simulink model "test"  (R2021a)
settings: Solver=VariableStepAuto  StartTime=0.0  StopTime=10.0  RelTol=1e-3
libraries: c2xlib x9
settings Model: EnablePacing=on  Creator=User  LastModifiedBy=User

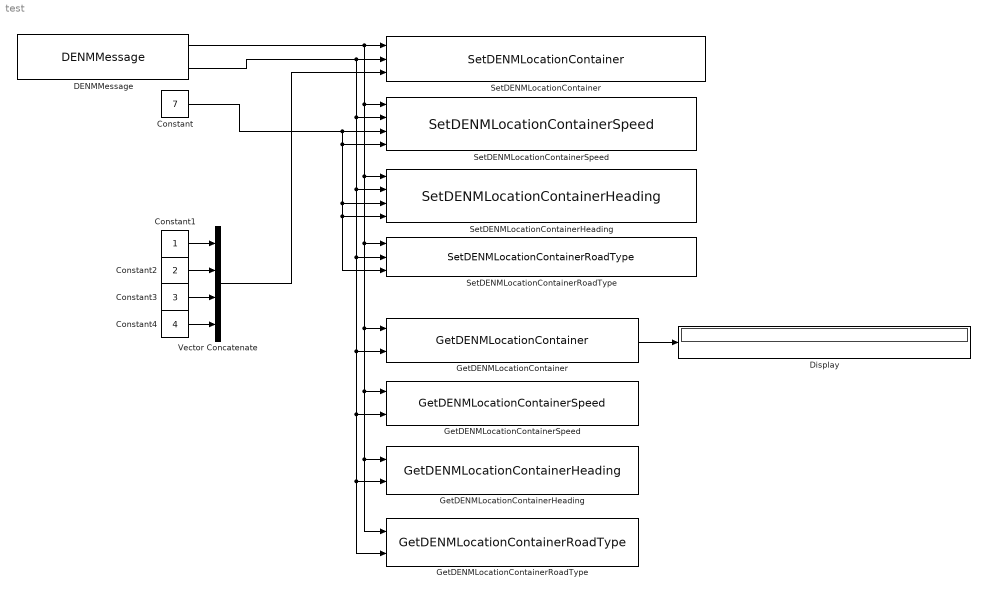
== system test ==
  Constant : Constant  Value=7
  Constant1 : Constant
  Constant2 : Constant  Value=2
  Constant3 : Constant  Value=3
  Constant4 : Constant  Value=4
  DENMMessage : c2xlib/DENMMessage  StationID=1  SequenceNumber=1  SimulateUsing=Code generation
      settings: SourceProductName=C2XLib
  Display : Display
  GetDENMLocationContainer : c2xlib/GetDENMLocationContainer  NumberTraces=1  TraceLength=1  SimulateUsing=Code generation
      settings: SourceProductName=C2XLib
  GetDENMLocationContainerHeading : c2xlib/GetDENMLocationContainerHeading  SimulateUsing=Code generation
      settings: SourceProductName=C2XLib
  GetDENMLocationContainerRoadType : c2xlib/GetDENMLocationContainerRoadType  SimulateUsing=Code generation
      settings: SourceProductName=C2XLib
  GetDENMLocationContainerSpeed : c2xlib/GetDENMLocationContainerSpeed  SimulateUsing=Code generation
      settings: SourceProductName=C2XLib
  SetDENMLocationContainer : c2xlib/SetDENMLocationContainer  NumberTraces=1  SimulateUsing=Code generation
      settings: SourceProductName=C2XLib
  SetDENMLocationContainerHeading : c2xlib/SetDENMLocationContainerHeading  SimulateUsing=Code generation
      settings: SourceProductName=C2XLib
  SetDENMLocationContainerRoadType : c2xlib/SetDENMLocationContainerRoadType  SimulateUsing=Code generation
      settings: SourceProductName=C2XLib
  SetDENMLocationContainerSpeed : c2xlib/SetDENMLocationContainerSpeed  SimulateUsing=Code generation
      settings: SourceProductName=C2XLib
  Vector Concatenate : Concatenate  NumInputs=4
  wires:
  Constant4/1 -> Vector Concatenate/4
  Constant3/1 -> Vector Concatenate/3
  Constant2/1 -> Vector Concatenate/2
  Constant1/1 -> Vector Concatenate/1
  DENMMessage/2 -> SetDENMLocationContainer/2, GetDENMLocationContainer/2, GetDENMLocationContainerSpeed/2, GetDENMLocationContainerRoadType/2, GetDENMLocationContainerHeading/2, SetDENMLocationContainerRoadType/2, SetDENMLocationContainerHeading/2, SetDENMLocationContainerSpeed/2
  Constant/1 -> SetDENMLocationContainerRoadType/3, SetDENMLocationContainerHeading/4, SetDENMLocationContainerHeading/3, SetDENMLocationContainerSpeed/4, SetDENMLocationContainerSpeed/3
  GetDENMLocationContainer/1 -> Display/1
  DENMMessage/1 -> SetDENMLocationContainer/1, GetDENMLocationContainer/1, GetDENMLocationContainerRoadType/1, GetDENMLocationContainerHeading/1, GetDENMLocationContainerSpeed/1, SetDENMLocationContainerRoadType/1, SetDENMLocationContainerHeading/1, SetDENMLocationContainerSpeed/1
  Vector Concatenate/1 -> SetDENMLocationContainer/3
